simulink model "rl_safety"  (R2021a)
settings: Solver=VariableStepAuto  StartTime=0.0  StopTime=inf  RelTol=1e-3
libraries: robotlib x7
settings Model: Creator=refulgent  LastModifiedBy=refulgent

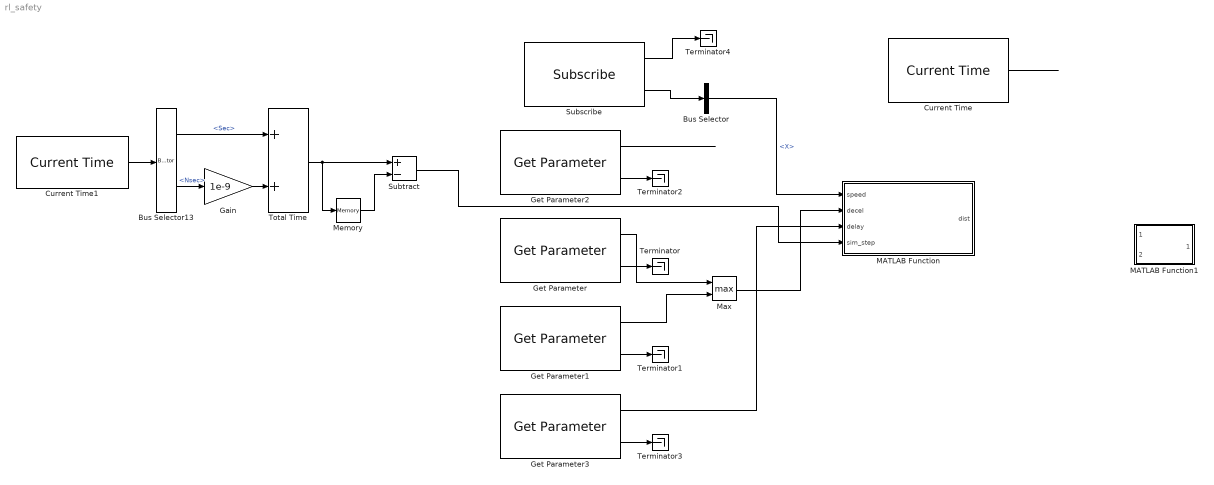
== system rl_safety ==
  Bus Selector : BusSelector  OutputSignals=Linear.X
  Bus Selector13 : BusSelector  OutputSignals=Sec,Nsec
  Current Time : robotlib/Current Time  OutputFormat=bus  SampleTime=-1  ModelName=robotlib
      settings: SourceProductBaseCode=RR
  Current Time1 : robotlib/Current Time  OutputFormat=bus  SampleTime=-1  ModelName=throttle_control
      settings: SourceProductBaseCode=RR
  Gain : Gain  Gain=1e-9
  Get Parameter : robotlib/Get Parameter  ParameterSource=Specify your own  ParameterName=max_decel  ParameterType=double  ParameterMaxArrayLength=16  ParameterInitialValue=4.6  SampleTime=-1  ShowErrorCodeOutput=on  ModelName=rl_safety  BlockId=ParamGet_rl_safety_1
      settings: SourceProductBaseCode=RR
  Get Parameter1 : robotlib/Get Parameter  ParameterSource=Specify your own  ParameterName=leadmax_decel  ParameterType=double  ParameterMaxArrayLength=16  ParameterInitialValue=4.6  SampleTime=-1  ShowErrorCodeOutput=on  ModelName=rl_safety  BlockId=ParamGet_rl_safety_3
      settings: SourceProductBaseCode=RR
  Get Parameter2 : robotlib/Get Parameter  ParameterSource=Specify your own  ParameterName=min_gap  ParameterType=double  ParameterMaxArrayLength=16  ParameterInitialValue=2.5  SampleTime=-1  ShowErrorCodeOutput=on  ModelName=rl_safety  BlockId=ParamGet_rl_safety_5
      settings: SourceProductBaseCode=RR
  Get Parameter3 : robotlib/Get Parameter  ParameterSource=Specify your own  ParameterName=delay  ParameterType=double  ParameterMaxArrayLength=16  ParameterInitialValue=0.0  SampleTime=-1  ShowErrorCodeOutput=on  ModelName=rl_safety  BlockId=ParamGet_rl_safety_8
      settings: SourceProductBaseCode=RR
  MATLAB Function : MATLAB Function  TreatAsAtomicUnit=on
  MATLAB Function1 : MATLAB Function  TreatAsAtomicUnit=on
  Max : MinMax  Function=max  Inputs=2
  Memory : Memory
  Subscribe : robotlib/Subscribe  topicSource=Specify your own  topic=leader_vel  messageType=geometry_msgs/Twist  SampleTime=-1  legacyBusStruct=off  messageQueueLength=1
  Subtract : Sum  Inputs=+-
  Terminator{,1..4} (5 alike) : Terminator
  Total Time : Sum
  wires:
  Get Parameter/2 -> Terminator/1
  Get Parameter1/2 -> Terminator1/1
  Get Parameter2/2 -> Terminator2/1
  Get Parameter3/2 -> Terminator3/1
  Get Parameter3/1 -> MATLAB Function/3(delay)
  Get Parameter/1 -> Max/1
  Get Parameter1/1 -> Max/2
  Max/1 -> MATLAB Function/2(decel)
  Get Parameter2/1 -> ?
  Subscribe/1 -> Terminator4/1
  Subscribe/2 -> Bus Selector/1
  Bus Selector/1 -> MATLAB Function/1(speed)  "<X>"
  Current Time/1 -> ?
  Gain/1 -> Total Time/2
  Total Time/1 -> Subtract/1, Memory/1
  Bus Selector13/1 -> Total Time/1  "<Sec>"
  Current Time1/1 -> Bus Selector13/1
  Bus Selector13/2 -> Gain/1  "<Nsec>"
  Memory/1 -> Subtract/2
  Subtract/1 -> MATLAB Function/4(sim_step)

== matlab function rl_safety/MATLAB Function1 ==
  data: brake_dist input; max_speed output; sim_step input
function max_speed = maximum_safe_stop_speed_euler(brake_dist, sim_step)

 if(brake_dist <=0)
     max_speed = 0.0;
     
 else
     speed_reduction = 4.*sim_step;
     
     sqrt_quantity = sqrt( (sim_step^2  + (4.0 * ( ( 
 end

== matlab function rl_safety/MATLAB Function ==
  data: speed input; dist output; decel input; delay input; sim_step input
function dist = brake_distance(speed, decel,  delay, sim_step)

speed_reduction = decel*sim_step;

steps_to_zero = int8(speed, speed_reduction);

dist = sim_step*( steps_to_zero*speed - speed_reduction*steps_to_zero*(steps_to_zero + 1) /2 ) + speed*delay;
